simulink model "PV_system_modified"  (R2024a)
settings: Solver=VariableStepAuto  StartTime=0  StopTime=1.2  RelTol=1e-3
InitFcn:
  | PV_system_par;
undefined symbols (not defined in the file): Clink, D1, Delta, F_LL, F_LLG, F_LLLG, F_SLG, Fc, Fnom, I, Increment_MPPT, Ki_Ireg, Ki_VDCreg, Kp_Ireg, Kp_VDCreg, L1, L2, LimitL_Ireg, LimitL_VDCreg, Limits_MPPT, LimitU_Ireg, LimitU_VDCreg, P_load, Pnom, Pnom_xfo, Qc_load, Ql_load, RL, RLff, Ts_Control, Ts_Power, Vf, Vfd, Vnom_dc, Vnom_prim, Vnom_sec
libraries: spsThreePhaseParallelRLCLoadLib x5, spsThreePhaseFaultLib x4, spsSeriesRLCBranchLib x3, spsThreePhaseVIMeasurementLib x3, spsPMUPLLBasedPositiveSequenceLib x3, spsThreePhaseBreakerLib x3, spsThreePhaseTransformerTwoWindingsLib x2, slpidlib x2, spsabctodq0Lib x2, spsPowerPositiveSequenceLib x2, spsVoltageMeasurementLib x2, spsThreePhaseSourceLib x1
settings Model: Creator=MathWorks  LastModifiedBy=745
settings SolverCC: AlgebraicLoopSolver=TrustRegion
settings DataIOCC: FinalStateName=xFinal236  InitialState=xFinal236  LimitDataPoints=on  SaveFinalState=on  SaveFormat=Array  SignalLoggingSaveFormat=ModelDataLogs  SaveOutput=off  SignalLogging=off  DSMLogging=off  SaveTime=off  ReturnWorkspaceOutputs=off
settings OptimizationCC: ExpressionDepthLimit=2147483647  LifeSpan=inf
settings DebuggingCC: UnderspecifiedInitializationDetection=Classic  MergeDetectMultiDrivingBlocksExec=none  SolverPrmCheckMsg=warning  FcnCallInpInsideContextMsg=warning  UnconnectedInputMsg=warning  UnconnectedOutputMsg=warning  UnconnectedLineMsg=warning  StateNameClashWarn=warning  SFUnexpectedBacktrackingDiag=warning  SFNoUnconditionalDefaultTransitionDiag=warning  SFExecutionAtInitializationDiag=none  ArithmeticOperatorsInVariantConditions=warning
settings HardwareCC: ProdBitPerPointer=32  ProdBitPerSizeT=32  ProdBitPerPtrDiffT=32  ProdLargestAtomicFloat=None  ProdIntDivRoundTo=Undefined  ProdEndianess=Unspecified  ProdWordSize=32  ProdHWDeviceType=32-bit Generic
settings ModelReferenceCC: EnableRefExpFcnMdlSchedulingChecks=on  PropagateSignalLabelsOutOfModel=off
settings SFSimCC: SimUseLocalCustomCode=off  CustomCodeUndefinedFunction=UseInterfaceOnly
settings RTWCC: RTWUseLocalCustomCode=off  GPUComputeCapability=3.5
settings CodeAppCC: StateflowObjectComments=on
settings GRTTargetCC: TargetLangStandard=C89/C90 (ANSI)  CombineOutputUpdateFcns=off  GRTInterface=on
settings ConfigComp: CovMetricSettings=dw  CovSaveCumulativeToWorkspaceVar=on  CovSaveSingleToWorkspaceVar=on  CovExternalEMLEnable=off  CovSFcnEnable=off
settings SimscapeCC: SimscapeNormalizeSystem=off

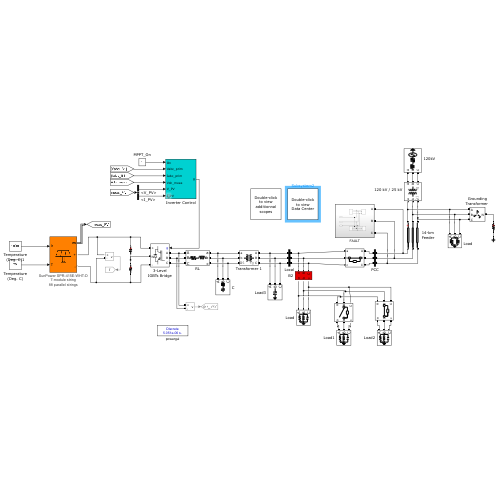
[thumbnail: Simulink's stored preview of the top-level diagram]
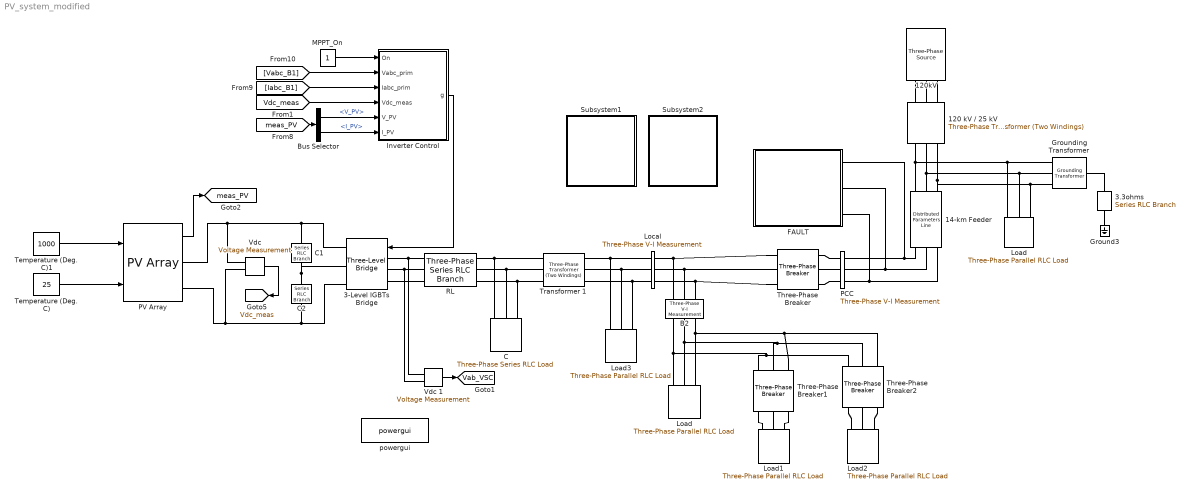
== system PV_system_modified ==
  " Load" : spsThreePhaseParallelRLCLoadLib/Three-Phase Parallel RLC Load  LConnTagsString=A|B|C  Configuration=Y (grounded)  NominalVoltage=Vnom_prim  Vabc=[1e3 1e3 1e3]  Vabcp=[1e3 1e3 1e3]  NominalFrequency=Fnom  UnbalancedPower=off  ActivePower=30e6  InductivePower=2e6  CapacitivePower=0  Pabc=[10e3 9e3 11e3]  QLabc=[100 90 110]  QCabc=[100 90 110]  Pabcp=[10e3 9e3 11e3]  QLabcp=[100 90 110]  QCabcp=[100 90 110]  Measurements=None  LoadType=constant Z
  "120 kV / 25 kV " : spsThreePhaseTransformerTwoWindingsLib/Three-Phase Transformer (Two Windings)  Winding1Connection=Yg  Winding2Connection=Delta (D1)  CoreType=Three single-phase transformers  SetSaturation=off  Hysteresis=off  DataFile='basic_model'  SetInitialFlux=off  Measurements=None  UNITS=pu  NominalPower=[47e6 Fnom ]  Winding1="[ 120e3  0.08/30   0.08 ]"  Winding2="[ Vnom_prim  0.08/30  0.08]"  Rm=500  Lm=500  L0=0.5  Saturation="[ 0,0  ;  0.005,1.2  ;  1.0,1.4 ]"  InitialFluxes=[ 0.8 , -0.8 , 0.7 ]  BreakLoop=off  DiscreteSolver=Trapezoidal iterative  DataType=off  TransfoNumber=0
  "120kV " : spsThreePhaseSourceLib/Three-Phase Source  InternalConnection=Yg  VoltagePhases=off  Voltage=(120000)*2.00543  PhaseAngle=-0.89585  Voltage_phases=[25e3 25e3 25e3]/sqrt(3)  PhaseAngles_phases=[0 -120 +120]  Frequency=Fnom  NonIdealSource=on  SpecifyImpedance=on  Resistance=0.8929  Inductance=16.58e-3  ShortCircuitLevel=2500e6  BaseVoltage=120e3  XRratio=7  BusType=swing  Pref=0  Qref=0  Prefabc=[10e3, 10e3, 10e3]  Qrefabc=[0, 0, 0]  Qmin=-inf  Qmax=inf
  14-km Feeder : spsDistributedParametersLineLib/Distributed Parameters Line  Phases=3  Length=14  Frequency=Fnom  Resistance=[0.1153 0.413]  Inductance=[1.05e-3 3.32e-3]  Capacitance=[11.33e-009 5.01e-009]  x1=[-6.06060606060606e-05 2.70356818258823e-09 -7448.2546576066 -48579.4518787537;-5.55555555555556e-05 2.70296987690159e-09 -7355.74615270988 -48593.5452588263;-5.05050505050505e-05 2.70236177241409e-09 -7263.21098177729 -48607.4624776782;-4.54545454545455e-05 2.70174387133024e-09 -7170.64948026713 -48621.2034848568;-4.04040404040404e-05 2.70111617589004e-09 -7078.06198373317 -48634.7682305481;-3.53535353535354e-05 2.70047868836901e-09 -6985.44882782342 -48648.1566655774;-3.03030303030303e-05 2.69983141107818e-09 -6892.81034827889 -48661.3687414089;-2.52525252525253e-05 2.69917434636406e-09 -6800.14688093242 -48674.4044101461;-2.02020202020202e-05 2.69850749660862e-09 -6707.45876170742 -48687.2636245322;-1.51515151515152e-05 2.69783086422934e-09 -6614.74632661666 -48699.94633795;-1.01010101010101e-05 2.69714445167914e-09 -6522.00991176108 -48712.4525044222;-5.05050505050505e-06 2.69644826144641e-09 -6429.24985332853 -48724.7820786115]  x2=[-6.06060606060606e-05 2.37344003803955e-09 -7561.18542903438 -48547.90625864;-5.55555555555556e-05 2.37275781583048e-09 -7468.73678212341 -48562.2147154482;-5.05050505050505e-05 2.37206699190463e-09 -7376.26105956317 -48576.3471246152;-4.54545454545455e-05 2.37136756876638e-09 -7283.75859659646 -48590.3034349081;-4.04040404040404e-05 2.37065954895129e-09 -7191.22972856301 -48604.0835957326;-3.53535353535354e-05 2.36994293502606e-09 -7098.67479089829 -48617.6875571329;-3.03030303030303e-05 2.36921772958855e-09 -7006.09411913227 -48631.115269792;-2.52525252525253e-05 2.36848393526779e-09 -6913.48804888821 -48644.3666850316;-2.02020202020202e-05 2.36774155472393e-09 -6820.85691588144 -48657.4417548129;-1.51515151515152e-05 2.36699059064823e-09 -6728.20105591817 -48670.340431736;-1.01010101010101e-05 2.3662310457631e-09 -6635.52080489422 -48683.0626690407;-5.05050505050505e-06 2.36546292282202e-09 -6542.81649879384 -48695.6084206065]  x3=[-6.06060606060606e-05 -1.40909290200934e-12 -26.0416127367686 -138.462500741439;-5.55555555555556e-05 -1.44156443022592e-12 -25.777933708129 -138.511832849198;-5.05050505050505e-05 -1.47403073248608e-12 -25.514161229377 -138.560662824145;-4.54545454545455e-05 -1.50649169109305e-12 -25.2502962567399 -138.60899048926;-4.04040404040404e-05 -1.53894718836944e-12 -24.9863397467807 -138.656815669347;-3.53535353535354e-05 -1.57139710665763e-12 -24.7222926563938 -138.704138191031;-3.03030303030303e-05 -1.60384132832025e-12 -24.4581559428022 -138.750957882757;-2.52525252525253e-05 -1.63627973574057e-12 -24.1939305635539 -138.797274574794;-2.02020202020202e-05 -1.66871221132296e-12 -23.929617476518 -138.843088099237;-1.51515151515152e-05 -1.70113863749325e-12 -23.6652176398819 -138.888398290001;-1.01010101010101e-05 -1.73355889669924e-12 -23.4007320121474 -138.933204982828;-5.05050505050505e-06 -1.76597287141107e-12 -23.1361615521271 -138.977508015286]  x4=[-6.06060606060606e-05 7.12180654461823e-12 -25.9634564564282 -178.876147541871;-5.55555555555556e-05 7.15742887638408e-12 -25.6228302123746 -178.925257586776;-5.05050505050505e-05 7.19302526105343e-12 -25.2821110804896 -178.973718992203;-4.54545454545455e-05 7.22859556958235e-12 -24.9413002959472 -179.021531582471;-4.04040404040404e-05 7.26413967302144e-12 -24.6003990942542 -179.068695184249;-3.53535353535354e-05 7.29965744251626e-12 -24.2594087112448 -179.115209626561;-3.03030303030303e-05 7.33514874930789e-12 -23.9183303830766 -179.161074740782;-2.52525252525253e-05 7.37061346473331e-12 -23.5771653462262 -179.206290360643;-2.02020202020202e-05 7.40605146022591e-12 -23.2359148374842 -179.250856322226;-1.51515151515152e-05 7.44146260731593e-12 -22.8945800939515 -179.294772463973;-1.01010101010101e-05 7.47684677763096e-12 -22.5531623530339 -179.338038626678;-5.05050505050505e-06 7.51220384289638e-12 -22.2116628524384 -179.380654653493]  x5=5.70973484498186e-05  V1=[0 0 0 2.512e-09 2.496e+04 2.496e+04;0 0 0 377 377 377;1.571 1.571 1.571 -1.525 -0.1391 -1.71]  V2=[0 0 0 2.184e-09 2.482e+04 2.482e+04;0 0 0 377 377 377;1.571 1.571 1.571 -1.563 -0.159 -1.73]  I1=[0 0 0 1.724e-11 7.342 7.342;0 0 0 377 377 377;1.571 1.571 1.571 0.451 3.099 1.528]  I2=[0 0 0 1.983e-11 170.2 170.2;0 0 0 377 377 377;1.571 1.571 1.571 -2.403 -0.1532 -1.724]  nHarmo=2  Measurements=None  Decoupling=off  VsMag0=0  VrMag0=0  VsAngle0=0  VrAngle0=0  IsMag0=0  IrMag0=0  IsAngle0=0  IrAngle0=0
      settings: LibrarySourceBlock=sps_lib/Power Grid Elements/Distributed Parameters Line
  3-Level IGBTs Bridge : spsThreeLevelBridgeLib/Three-Level Bridge  Arms=3  SnubberResistance=Rs  SbubberCapacitance=Cs  Device=IGBT / Diodes  Ron=Ron  ForwardVoltages="[  Vfd  Vf ]"  Measurements=None
      settings: AttributesFormatString=\n  LibrarySourceBlock=sps_lib/Power Electronics/Three-Level Bridge
  "3.3ohms " : spsSeriesRLCBranchLib/Series RLC Branch  LConnTagsString=__new0  RConnTagsString=__new0  BranchType=R  Resistance=3.3  Inductance=[]  SetiL0=off  InitialCurrent=0  Capacitance=[]  Setx0=off  InitialVoltage=0  Measurements=None
  B2 : spsThreePhaseVIMeasurementLib/Three-Phase V-I Measurement  VoltageMeasurement=phase-to-ground  SetLabelV=on  LabelV=Vabc_Load  Vpu=on  VpuLL=off  CurrentMeasurement=yes  SetLabelI=on  LabelI=Iabc_Load  Ipu=on  Pbase=250e3  Vbase=25e3  OutputType=Magnitude  PhasorSimulation=off  PSBequivalent=0
  Bus Selector : BusSelector  OutputSignals=V_PV,I_PV
  C : spsThreePhaseSeriesRLCLoadLib/Three-Phase Series RLC Load  LConnTagsString=A|B|C  Configuration=Delta  NominalVoltage=Vnom_sec  Vabc=[1e3 1e3 1e3]  Vabcp=[1e3 1e3 1e3]  NominalFrequency=Fnom  UnbalancedPower=off  ActivePower=Pc  InductivePower=0  CapacitivePower=Qc  Pabc=[10e3 9e3 11e3]  QLabc=[100 90 110]  QCabc=[100 90 110]  Pabcp=[10e3 9e3 11e3]  QLabcp=[100 90 110]  QCabcp=[100 90 110]  Measurements=None  LoadType=constant Z
  C1 : spsSeriesRLCBranchLib/Series RLC Branch  LConnTagsString=__new0  RConnTagsString=__new0  BranchType=C  Resistance=1.0  Inductance=1.0  SetiL0=off  InitialCurrent=0  Capacitance=Clink  Setx0=on  InitialVoltage=Vnom_dc/2  Measurements=None
  C2 : spsSeriesRLCBranchLib/Series RLC Branch  LConnTagsString=__new0  RConnTagsString=__new0  BranchType=C  Resistance=1.0  Inductance=1.0  SetiL0=off  InitialCurrent=0  Capacitance=Clink  Setx0=on  InitialVoltage=Vnom_dc/2  Measurements=None
  FAULT : Subsystem
  Ground3 : spsGroundLib/Ground  LConnTagsString=a
  "Grounding Transformer " : spsGroundingTransformerLib/Grounding Transformer   UNITS=pu  NominalPower="[100e6   Fnom]"  NominalVoltage=Vnom_prim  ZeroSequenceImpedance_pu=[0.025 0.75]  MagnetizationBranch_pu=[500 500]  ZeroSequenceImpedance_SI=[0.052083 589.05]  MagnetizationBranch_SI=[1041.7 3.927e+005]  Measurements=None
      settings: LibrarySourceBlock=|
      | sps_lib/Power Grid Elements/Grounding
      | Transformer
  Inverter Control : Subsystem  mask(Inverter Control){Pnom=Pnom, Fnom=Fnom, Vnom_prim=Vnom_prim, Vnom_sec=Vnom_sec, Vnom_dc=Vnom_dc, Increment_MPPT=Increment_MPPT, Limits_MPPT=Limits_MPPT, Vdc_ref_Init=Vnom_dc, Kp_VDCreg=Kp_VDCreg, Ki_VDCreg=Ki_VDCreg, Kp_Ireg=Kp_Ireg, Ki_Ireg=Ki_Ireg, RLff=RLff, Fc=Fc, Ts_Control=Ts_Control, Ts_PWMgenerator=Ts_Power}
      mask prompts: Pnom "Power (VA)"; Fnom "Frequency (Hz)"; Vnom_prim "Primary voltage (Vrms LL)"; Vnom_sec "Secondary voltage (Vrms LL)"; Vnom_dc "DC voltage (V)"; Increment_MPPT "Output increment (V)"; Limits_MPPT "Output limits [ Upper  Lower ]"; Vdc_ref_Init "Output initial value (V)"; Kp_VDCreg "Proportional gain"; Ki_VDCreg "Integral gain"; Kp_Ireg "Proportional gain"; Ki_Ireg "Integral gain"; RLff "Feedforward Values [Rff Lff]"; Fc "Carrier frequency (Hz)"; Ts_Control "Control systems"; Ts_PWMgenerator "PWM generator"
      mask help:
      | The main components of the Inverter Control are:
      | 1. PLL & Measurements
      | 2. Maximum Power Point Tracker System (MPPT) using a Perturb & Observe algorithm
      | 3. DC Voltage Regulator
      | 4. Current Regulator
      | 5. PWM Modulator
      mask DialogControl Container4 Prompt: Nominal Values:
      mask DialogControl Container3 Prompt: MPPT Controller:
      mask DialogControl Container8 Prompt: Dc Voltage Regulator:
      mask DialogControl Container6 Prompt: Current Regulator:
      mask DialogControl Container9 Prompt: PWM Modulator:
      mask DialogControl SampleTimes Prompt: Sample Times:
  Load : spsThreePhaseParallelRLCLoadLib/Three-Phase Parallel RLC Load  LConnTagsString=A|B|C  Configuration=Y (grounded)  NominalVoltage=Vnom_prim  Vabc=[1e3 1e3 1e3]  Vabcp=[1e3 1e3 1e3]  NominalFrequency=Fnom  UnbalancedPower=off  ActivePower=P_load*0.75  InductivePower=Ql_load*0.75  CapacitivePower=Qc_load*0.75  Pabc=[10e3 9e3 11e3]  QLabc=[100 90 110]  QCabc=[100 90 110]  Pabcp=[10e3 9e3 11e3]  QLabcp=[100 90 110]  QCabcp=[100 90 110]  Measurements=None  LoadType=constant Z
  Load1 : spsThreePhaseParallelRLCLoadLib/Three-Phase Parallel RLC Load  LConnTagsString=A|B|C  Configuration=Y (grounded)  NominalVoltage=Vnom_prim  Vabc=[1e3 1e3 1e3]  Vabcp=[1e3 1e3 1e3]  NominalFrequency=Fnom  UnbalancedPower=off  ActivePower=P_load*0.25  InductivePower=Ql_load*0.25  CapacitivePower=Qc_load*0.25  Pabc=[10e3 9e3 11e3]  QLabc=[100 90 110]  QCabc=[100 90 110]  Pabcp=[10e3 9e3 11e3]  QLabcp=[100 90 110]  QCabcp=[100 90 110]  Measurements=None  LoadType=constant Z
  Load2 : spsThreePhaseParallelRLCLoadLib/Three-Phase Parallel RLC Load  LConnTagsString=A|B|C  Configuration=Y (grounded)  NominalVoltage=Vnom_prim  Vabc=[1e3 1e3 1e3]  Vabcp=[1e3 1e3 1e3]  NominalFrequency=Fnom  UnbalancedPower=off  ActivePower=P_load*0.25  InductivePower=Ql_load*0.25  CapacitivePower=Qc_load*0.25  Pabc=[10e3 9e3 11e3]  QLabc=[100 90 110]  QCabc=[100 90 110]  Pabcp=[10e3 9e3 11e3]  QLabcp=[100 90 110]  QCabcp=[100 90 110]  Measurements=None  LoadType=constant Z
  Load3 : spsThreePhaseParallelRLCLoadLib/Three-Phase Parallel RLC Load  LConnTagsString=A|B|C  Configuration=Y (grounded)  NominalVoltage=Vnom_prim  Vabc=[1e3 1e3 1e3]  Vabcp=[1e3 1e3 1e3]  NominalFrequency=Fnom  UnbalancedPower=off  ActivePower=0  InductivePower=0  CapacitivePower=1  Pabc=[10e3 9e3 11e3]  QLabc=[100 90 110]  QCabc=[100 90 110]  Pabcp=[10e3 9e3 11e3]  QLabcp=[100 90 110]  QCabcp=[100 90 110]  Measurements=None  LoadType=constant Z
  Local : spsThreePhaseVIMeasurementLib/Three-Phase V-I Measurement  VoltageMeasurement=phase-to-ground  SetLabelV=on  LabelV=Vabc_Local  Vpu=on  VpuLL=off  CurrentMeasurement=yes  SetLabelI=on  LabelI=Iabc_Local  Ipu=on  Pbase=250e3  Vbase=25e3  OutputType=Magnitude  PhasorSimulation=off  PSBequivalent=0
  MPPT_On : Constant
  PCC : spsThreePhaseVIMeasurementLib/Three-Phase V-I Measurement  VoltageMeasurement=phase-to-ground  SetLabelV=on  LabelV=Vabc_PCC  Vpu=on  VpuLL=off  CurrentMeasurement=yes  SetLabelI=on  LabelI=Iabc_PCC  Ipu=on  Pbase=250e3  Vbase=25e3  OutputType=Magnitude  PhasorSimulation=off  PSBequivalent=0
  PV Array : spsPVArrayLib/PV Array  Npar=88  Nser=7  PlotType=array @ 1000 W/m2 & specified temperatures  S_vec="[ 1000  500  100 ]"  Temp_C_vec="[ 45 25  ]"  ModuleName=SunPower SPR-415E-WHT-D  PlotWhenSelected=off  Pm=414.801  Ncell=128  Voc=85.3  Isc=6.09  Vm=72.9  Im=5.69  beta_Voc_pc=-0.229  alpha_Isc_pc=0.030706  beta_Voc=-0.19534  alpha_Isc=0.00187  IL=6.0978  I0=7.1698e-13  nI=0.87223  Rsh=419.7781  Rs=0.53711  RobustModel=off  RobustCellTemperature=25  BAL=on  Tc=1e-6  Tfilter=5e-5
      settings: AttributesFormatString=|
      | %<ModuleName>
      | %<Nser>-module string
      | %<Npar> parallel strings
  RL : spsThreePhaseSeriesRLCBranchLib/Three-Phase Series RLC Branch  LConnTagsString=A|B|C  RConnTagsString=A|B|C  BranchType=RL  Resistance=RL(1)  Inductance=RL(2)  Capacitance=inf  Measurements=None
  Subsystem1 : Subsystem
      mask Display: disp('Double-click\nto view\nadditionnal\nscopes')
  Subsystem2 : Subsystem
      mask Display: disp('Double-click\nto view\nData Center')
  Temperature (Deg. C) : Constant  Value=25
  Temperature (Deg. C)1 : Constant  Value=1000
  Three-Phase Breaker : spsThreePhaseBreakerLib/Three-Phase Breaker  InitialState=closed  SwitchA=on  SwitchB=on  SwitchC=on  SwitchTimes=[0.5+I 1.5+I]  External=off  BreakerResistance=0.01  SnubberResistance=1e6  SnubberCapacitance=inf  Measurements=None
  Three-Phase Breaker1 : spsThreePhaseBreakerLib/Three-Phase Breaker  InitialState=open  SwitchA=on  SwitchB=on  SwitchC=on  SwitchTimes=[0.5+L1 1.5+L1]  External=off  BreakerResistance=0.01  SnubberResistance=1e6  SnubberCapacitance=inf  Measurements=None
  Three-Phase Breaker2 : spsThreePhaseBreakerLib/Three-Phase Breaker  InitialState=closed  SwitchA=on  SwitchB=on  SwitchC=on  SwitchTimes=[0.5+L2 1.5+L2]  External=off  BreakerResistance=0.01  SnubberResistance=1e6  SnubberCapacitance=inf  Measurements=None
  Transformer 1 : spsThreePhaseTransformerTwoWindingsLib/Three-Phase Transformer (Two Windings)  Winding1Connection=Yg  Winding2Connection=Delta (D1)  CoreType=Three single-phase transformers  SetSaturation=off  Hysteresis=off  DataFile='hysteresis'  SetInitialFlux=off  Measurements=None  UNITS=pu  NominalPower=[Pnom_xfo, Fnom ]  Winding1=W1_xfo  Winding2=W2_xfo  Rm=Rm_xfo  Lm=Lm_xfo  L0=0.5  Saturation=[ 0,0 ; 0.0024,1.2 ; 1.0,1.52 ]  InitialFluxes=[ 0.8 , -0.8 , 0.7 ]  BreakLoop=off  DiscreteSolver=Trapezoidal iterative  DataType=off  TransfoNumber=0
  "Vdc " : spsVoltageMeasurementLib/Voltage Measurement  Tag=PoWeRsYsTeMmEaSuReMeNt  PhasorSimulation=off  OutputType=Magnitude  PSBequivalent=0
  Vdc 1 : spsVoltageMeasurementLib/Voltage Measurement  Tag=PoWeRsYsTeMmEaSuReMeNt  PhasorSimulation=off  OutputType=Magnitude  PSBequivalent=0
  powergui : sps_lib/powergui  Priority=1  SimulationMode=Discrete  SampleTime=Ts_Power  frequency=60  Iterations=50  frequencyindice=0  Pbase=100e6  ErrMax=0.0001  UnitsV=kV  UnitsW=MW  buscounter=0  FunctionMessages=off  echomessages=off  EnableUseOfTLC=off  CurrentSourceSwitches=off  DisableSnubberDevices=off  DisableRonSwitches=off  DisableVfSwitches=off  DisplayEquations=off  AutomaticDiscreteSolvers=off  SolverType=Tustin  Interpol=off  ExternalGateDelay=off  methode=off  Ts=0  x0status=blocks  SPID=off  SwTol=0  HookPort=off  NonlinearTolerance=1e-4  nMaxIteration=15  ContinueOnMaxIteration=off  RestoreLinks=warning  ResistiveCurrentMeasurement=off  Frange=[0:2:500]  Ylog=off  Xlog=on  ShowGrid=off  save=off  variable=ZData  structure=VaIa_Grid  ZoomFFT=off  StartTime=1.4  cycles=3  DisplayStyle=1  fundamental=60  FreqAxis=on  MaxFrequency=5000  frequencyindicesteady=1  RmsSteady=1  display=off
  tag scope: Vab_VSC=global, Vdc_meas=global, meas_PV=global
  wires:
  Vdc 1/1 -> [Vab_VSC]
  PV Array/1 -> [meas_PV]
  Inverter Control/1(g) -> 3-Level IGBTs Bridge/1
  [Vabc_B1] -> Inverter Control/2(Vabc_prim)
  [Iabc_B1] -> Inverter Control/3(Iabc_prim)
  [Vdc_meas] -> Inverter Control/4(Vdc_meas)
  [meas_PV] -> Bus Selector/1
  "Vdc "/1 -> [Vdc_meas]
  Bus Selector/1 -> Inverter Control/5(V_PV)  "<V_PV>"
  Bus Selector/2 -> Inverter Control/6(I_PV)  "<I_PV>"
  MPPT_On/1 -> Inverter Control/1(On)
  Temperature (Deg. C)/1 -> PV Array/2
  Temperature (Deg. C)1/1 -> PV Array/1
  connections:
  Local/LConn1 -- Load3/LConn1 -- Transformer 1/LConn1
  Local/LConn2 -- Load3/LConn2 -- Transformer 1/LConn2
  Local/LConn3 -- Transformer 1/LConn3 -- Load3/LConn3
  C2/LConn1 -- 3-Level IGBTs Bridge/RConn2 -- C1/RConn1
  C1/LConn1 -- PV Array/RConn1 -- "Vdc "/LConn1 -- 3-Level IGBTs Bridge/RConn1
  C2/RConn1 -- PV Array/RConn2 -- "Vdc "/LConn2 -- 3-Level IGBTs Bridge/RConn3
  RL/LConn1 -- Vdc 1/LConn1 -- 3-Level IGBTs Bridge/LConn1
  RL/LConn2 -- Vdc 1/LConn2 -- 3-Level IGBTs Bridge/LConn2
  RL/LConn3 -- 3-Level IGBTs Bridge/LConn3
  C/LConn1 -- Transformer 1/RConn1 -- RL/RConn1
  C/LConn2 -- Transformer 1/RConn2 -- RL/RConn2
  C/LConn3 -- Transformer 1/RConn3 -- RL/RConn3
  "Grounding Transformer "/RConn1 -- "3.3ohms "/LConn1
  "3.3ohms "/RConn1 -- Ground3/LConn1
  "120 kV / 25 kV "/RConn1 -- 14-km Feeder/LConn1 -- " Load"/LConn1 -- "Grounding Transformer "/LConn1
  "120 kV / 25 kV "/RConn2 -- " Load"/LConn2 -- "Grounding Transformer "/LConn2 -- 14-km Feeder/LConn2
  "120 kV / 25 kV "/RConn3 -- " Load"/LConn3 -- "Grounding Transformer "/LConn3 -- 14-km Feeder/LConn3
  "120kV "/RConn1 -- "120 kV / 25 kV "/LConn1
  "120kV "/RConn2 -- "120 kV / 25 kV "/LConn2
  "120kV "/RConn3 -- "120 kV / 25 kV "/LConn3
  B2/LConn1 -- Local/RConn1 -- Three-Phase Breaker/RConn1
  Load/LConn2 -- Three-Phase Breaker2/LConn2 -- Three-Phase Breaker1/LConn2 -- B2/RConn2
  B2/RConn1 -- Three-Phase Breaker2/LConn1 -- Three-Phase Breaker1/LConn1 -- Load/LConn1
  Load/LConn3 -- Three-Phase Breaker2/LConn3 -- Three-Phase Breaker1/LConn3 -- B2/RConn3
  Local/RConn2 -- Three-Phase Breaker/RConn2 -- B2/LConn2
  Local/RConn3 -- Three-Phase Breaker/RConn3 -- B2/LConn3
  Three-Phase Breaker1/RConn3 -- Load1/LConn3
  Three-Phase Breaker1/RConn2 -- Load1/LConn2
  Three-Phase Breaker1/RConn1 -- Load1/LConn1
  Load2/LConn1 -- Three-Phase Breaker2/RConn1
  Load2/LConn2 -- Three-Phase Breaker2/RConn2
  Load2/LConn3 -- Three-Phase Breaker2/RConn3
  PCC/LConn2 -- Three-Phase Breaker/LConn2
  PCC/LConn1 -- Three-Phase Breaker/LConn1
  PCC/LConn3 -- Three-Phase Breaker/LConn3
  14-km Feeder/RConn1 -- PCC/RConn1 -- FAULT/LConn1
  14-km Feeder/RConn2 -- PCC/RConn2 -- FAULT/LConn2
  14-km Feeder/RConn3 -- FAULT/LConn3 -- PCC/RConn3

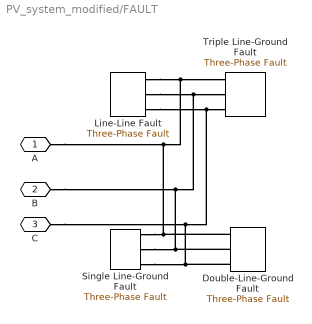
== system PV_system_modified/FAULT ==
  Double-Line-Ground Fault : spsThreePhaseFaultLib/Three-Phase Fault  InitialStates=0  FaultA=on  FaultB=on  FaultC=off  GroundFault=on  SwitchTimes=[0.5+F_LLG 0.6+F_LLG]  External=off  SwitchStatus=NaN  FaultResistance=Rf  GroundResistance=Rg  SnubberResistance=1e6  SnubberCapacitance=inf  Measurements=None
  Line-Line Fault : spsThreePhaseFaultLib/Three-Phase Fault  InitialStates=0  FaultA=on  FaultB=on  FaultC=off  GroundFault=off  SwitchTimes=[0.5+F_LL 0.6+F_LL]  External=off  SwitchStatus=NaN  FaultResistance=Rf  GroundResistance=0.01  SnubberResistance=1e6  SnubberCapacitance=inf  Measurements=None
  Single Line-Ground Fault : spsThreePhaseFaultLib/Three-Phase Fault  InitialStates=0  FaultA=on  FaultB=off  FaultC=off  GroundFault=on  SwitchTimes=[0.5+F_SLG 0.6+F_SLG]  External=off  SwitchStatus=NaN  FaultResistance=Rf  GroundResistance=Rg  SnubberResistance=1e6  SnubberCapacitance=inf  Measurements=None
  Triple Line-Ground Fault : spsThreePhaseFaultLib/Three-Phase Fault  InitialStates=0  FaultA=on  FaultB=on  FaultC=on  GroundFault=on  SwitchTimes=[0.5+F_LLLG 0.6+F_LLLG]  External=off  SwitchStatus=NaN  FaultResistance=Rf  GroundResistance=Rg  SnubberResistance=1e6  SnubberCapacitance=inf  Measurements=None
  A : PMIOPort  Side=Left
  B : PMIOPort  Port=2  Side=Left
  C : PMIOPort  Port=3  Side=Left
  connections:
  Line-Line Fault/LConn1 -- Double-Line-Ground Fault/LConn1 -- Single Line-Ground Fault/LConn1 -- A/RConn1 -- Triple Line-Ground Fault/LConn1
  Line-Line Fault/LConn2 -- Double-Line-Ground Fault/LConn2 -- Single Line-Ground Fault/LConn2 -- B/RConn1 -- Triple Line-Ground Fault/LConn2
  Line-Line Fault/LConn3 -- Double-Line-Ground Fault/LConn3 -- Single Line-Ground Fault/LConn3 -- C/RConn1 -- Triple Line-Ground Fault/LConn3

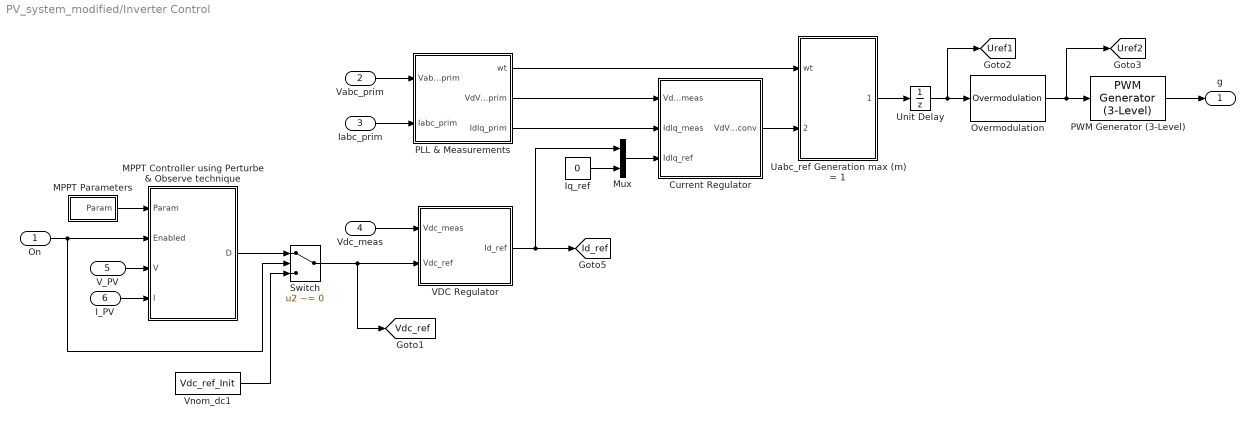
== system PV_system_modified/Inverter Control ==
  On : Inport  PortDimensions=1
  Vabc_prim : Inport  Port=2  PortDimensions=3
  Iabc_prim : Inport  Port=3  PortDimensions=3
  Vdc_meas : Inport  Port=4  PortDimensions=1
  V_PV : Inport  Port=5  PortDimensions=1
  I_PV : Inport  Port=6  PortDimensions=1
  Current Regulator : Subsystem
  Iq_ref : Constant  Value=0
  MPPT Parameters : Subsystem
  "MPPT Controller using Perturbe & Observe technique " : MATLAB Function  TreatAsAtomicUnit=on
  Mux : Mux  Inputs=2
  Overmodulation : spsOvermodulationLib/Overmodulation  OverModType=Flat top
      settings: LibrarySourceBlock=sps_lib/Power Electronics/Power Electronics Control/Overmodulation
  PLL & Measurements : Subsystem
  PWM Generator (3-Level) : spsPWMGenerator3LevelLib/PWM Generator (3-Level)  ModulatorType=Three-phase bridge (12 pulses)  ModulatorMode=Unsynchronized  nF=27  Fc=Fc  ModulatingSignals=off  m=0.8  Freq=60  Phase=0  Ts=Ts_PWMgenerator
      settings: LibrarySourceBlock=|
      | sps_lib/Power Electronics/Power Electronics Control/PWM Generator
      | (3-Level)
  Switch : Switch  Criteria=u2 ~= 0  SaturateOnIntegerOverflow=off  InputSameDT=off
  Uabc_ref Generation max (m) = 1 : Subsystem
  Unit Delay : UnitDelay  SampleTime=Ts_Control  HasFrameUpgradeWarning=on
  VDC Regulator : Subsystem
  Vnom_dc1 : Constant  Value=Vdc_ref_Init
  g : Outport  VectorParamsAs1DForOutWhenUnconnected=off
  tag scope: Id_ref=global, Uref1=global, Uref2=global, Vdc_ref=global
  wires:
  PLL & Measurements/1(wt) -> Uabc_ref Generation max (m) = 1/1(wt)
  Current Regulator/1(VdVq_conv) -> Uabc_ref Generation max (m) = 1/2(VdVq_conv)
  Iq_ref/1 -> Mux/2
  Mux/1 -> Current Regulator/3(IdIq_ref)
  PLL & Measurements/3(IdIq_prim) -> Current Regulator/2(IdIq_meas)
  PLL & Measurements/2(VdVq_prim) -> Current Regulator/1(VdVq_meas)
  Vabc_prim/1 -> PLL & Measurements/1(Vabc_prim)
  Iabc_prim/1 -> PLL & Measurements/2(Iabc_prim)
  PWM Generator (3-Level)/1 -> g/1
  Vdc_meas/1 -> VDC Regulator/1(Vdc_meas)
  VDC Regulator/1(Id_ref) -> [Id_ref], Mux/1
  V_PV/1 -> "MPPT Controller using Perturbe & Observe technique "/3(V)
  I_PV/1 -> "MPPT Controller using Perturbe & Observe technique "/4(I)
  MPPT Parameters/1(Param) -> "MPPT Controller using Perturbe & Observe technique "/1(Param)
  On/1 -> "MPPT Controller using Perturbe & Observe technique "/2(Enabled), Switch/2
  Overmodulation/1 -> [Uref2], PWM Generator (3-Level)/1
  Unit Delay/1 -> [Uref1], Overmodulation/1
  "MPPT Controller using Perturbe & Observe technique "/1(D) -> Switch/1
  Switch/1 -> [Vdc_ref], VDC Regulator/2(Vdc_ref)
  Vnom_dc1/1 -> Switch/3
  Uabc_ref Generation max (m) = 1/1(Uabc_ref) -> Unit Delay/1

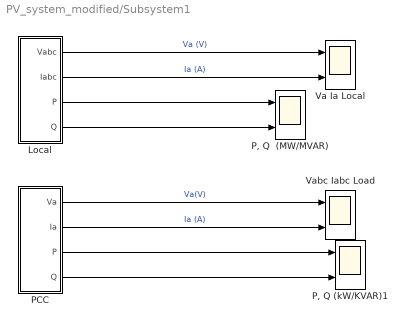
== system PV_system_modified/Subsystem1 ==
  Local : Subsystem
  "P, Q  (MW/MVAR)" : Scope  NumInputPorts=2
  "P, Q (kW/KVAR)1" : Scope  NumInputPorts=2
  PCC : Subsystem
  Va Ia Local : Scope  NumInputPorts=2
  Vabc Iabc Load : Scope  NumInputPorts=2
  wires:
  Local/3(P) -> "P, Q  (MW/MVAR)"/1
  Local/1(Vabc) -> Va Ia Local/1  "Va (V)"
  PCC/2(Ia) -> Vabc Iabc Load/2  "Ia (A)"
  PCC/4(Q) -> "P, Q (kW/KVAR)1"/2
  PCC/3(P) -> "P, Q (kW/KVAR)1"/1
  PCC/1(Va) -> Vabc Iabc Load/1  "Va(V)"
  Local/2(Iabc) -> Va Ia Local/2  "Ia (A)"
  Local/4(Q) -> "P, Q  (MW/MVAR)"/2

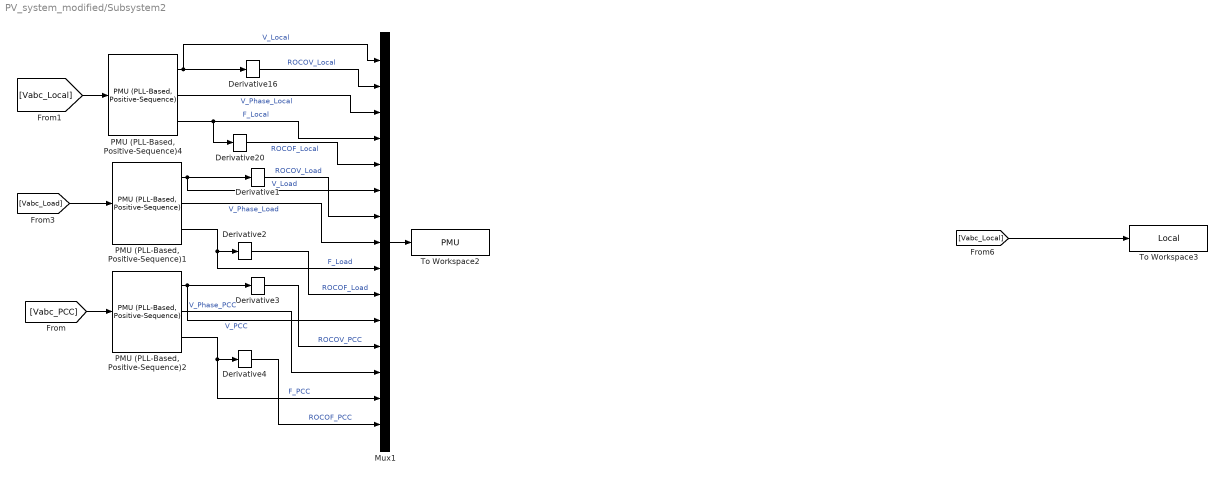
== system PV_system_modified/Subsystem2 ==
  Derivative{1..4,16,20} (6 alike) : Derivative
  Mux1 : Mux  Inputs=15
  "PMU (PLL-Based, Positive-Sequence)1" : spsPMUPLLBasedPositiveSequenceLib/PMU (PLL-Based, Positive-Sequence)  nominalFrequency=60  samplingRate=64  reportingFactor=1
      settings: LibrarySourceBlock=|
      | sps_lib/Sensors and Measurements/PMU
      | (PLL-Based,
      | Positive-Sequence)
  "PMU (PLL-Based, Positive-Sequence)2" : spsPMUPLLBasedPositiveSequenceLib/PMU (PLL-Based, Positive-Sequence)  nominalFrequency=60  samplingRate=64  reportingFactor=1
      settings: LibrarySourceBlock=|
      | sps_lib/Sensors and Measurements/PMU
      | (PLL-Based,
      | Positive-Sequence)
  "PMU (PLL-Based, Positive-Sequence)4" : spsPMUPLLBasedPositiveSequenceLib/PMU (PLL-Based, Positive-Sequence)  nominalFrequency=60  samplingRate=64  reportingFactor=1
      settings: LibrarySourceBlock=|
      | sps_lib/Sensors and Measurements/PMU
      | (PLL-Based,
      | Positive-Sequence)
  To Workspace2 : ToWorkspace  VariableName=PMU  SampleTime=1/60
      settings: Save2DSignal=2-D array (concatenate along first dimension)
  To Workspace3 : ToWorkspace  VariableName=Local  SampleTime=1/60/64
      settings: Save2DSignal=2-D array (concatenate along first dimension)
  wires:
  Derivative16/1 -> Mux1/2  "ROCOV_Local"
  "PMU (PLL-Based, Positive-Sequence)4"/1 -> Mux1/1, Derivative16/1  "V_Local"
  Mux1/1 -> To Workspace2/1
  "PMU (PLL-Based, Positive-Sequence)4"/2 -> Mux1/3  "V_Phase_Local"
  "PMU (PLL-Based, Positive-Sequence)4"/3 -> Mux1/4, Derivative20/1  "F_Local"
  Derivative20/1 -> Mux1/5  "ROCOF_Local"
  [Vabc_Local] -> "PMU (PLL-Based, Positive-Sequence)4"/1
  [Vabc_Local] -> To Workspace3/1
  [Vabc_Load] -> "PMU (PLL-Based, Positive-Sequence)1"/1
  Derivative2/1 -> Mux1/10  "ROCOF_Load"
  "PMU (PLL-Based, Positive-Sequence)1"/3 -> Mux1/9, Derivative2/1  "F_Load"
  "PMU (PLL-Based, Positive-Sequence)1"/2 -> Mux1/8  "V_Phase_Load"
  "PMU (PLL-Based, Positive-Sequence)1"/1 -> Mux1/6, Derivative1/1  "V_Load"
  Derivative1/1 -> Mux1/7  "ROCOV_Load"
  Derivative3/1 -> Mux1/12  "ROCOV_PCC"
  "PMU (PLL-Based, Positive-Sequence)2"/1 -> Mux1/11, Derivative3/1  "V_PCC"
  "PMU (PLL-Based, Positive-Sequence)2"/2 -> Mux1/13  "V_Phase_PCC"
  "PMU (PLL-Based, Positive-Sequence)2"/3 -> Mux1/14, Derivative4/1  "F_PCC"
  Derivative4/1 -> Mux1/15  "ROCOF_PCC"
  [Vabc_PCC] -> "PMU (PLL-Based, Positive-Sequence)2"/1

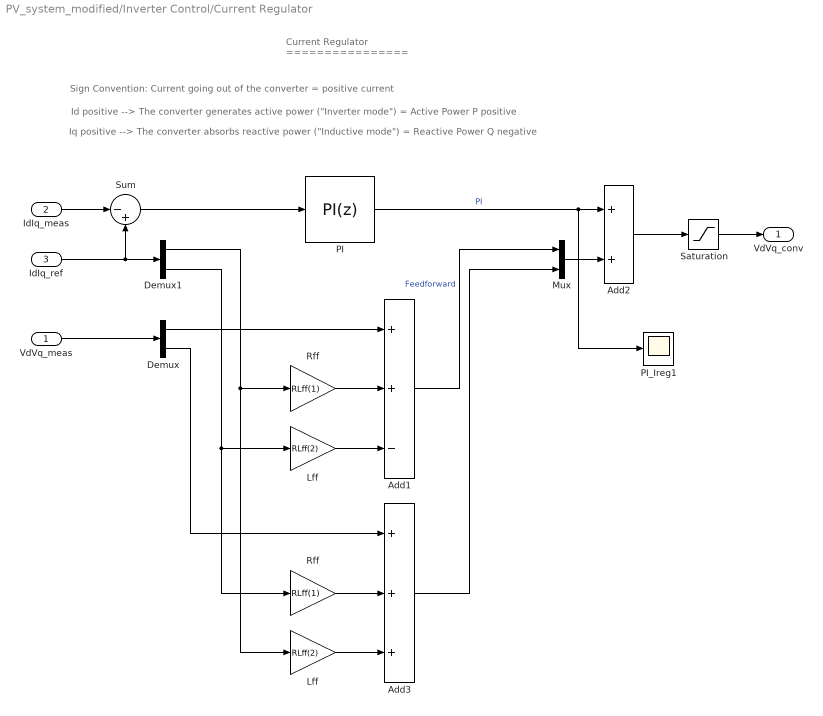
== system PV_system_modified/Inverter Control/Current Regulator ==
  note: Current Regulator
      | ================
  note: Sign Convention: Current going out of the converter = positive current
  note: Iq positive --> The converter absorbs reactive power ("Inductive mode") = Reactive Power Q negative
  note: Id positive --> The converter generates active power ("Inverter mode") = Active Power P positive
  VdVq_meas : Inport  PortDimensions=2
  IdIq_meas : Inport  Port=2  PortDimensions=2
  IdIq_ref : Inport  Port=3  PortDimensions=2
  Add1 : Sum  Inputs=++-
  Add2 : Sum
  Add3 : Sum  Inputs=+++
  Demux : Demux  Outputs=2
  Demux1 : Demux  Outputs=2
  Lff : Gain  Gain=RLff(2)  SaturateOnIntegerOverflow=on  OutDataTypeStr=Inherit: Same as input  ParamDataTypeStr=Inherit: Same as input
  "Lff  " : Gain  Gain=RLff(2)  SaturateOnIntegerOverflow=on  OutDataTypeStr=Inherit: Same as input  ParamDataTypeStr=Inherit: Same as input
  Mux : Mux  Inputs=2
  PI : slpidlib/PID Controller  Controller=PI  Form=Parallel  TimeDomain=Discrete-time  UseExternalTs=off  SampleTime=Ts_Control  IntegratorMethod=Forward Euler  FilterMethod=Forward Euler  ControllerParametersSource=internal  P=Kp_Ireg  I=Ki_Ireg  UseKiTs=off  D=0  UseExternalDerivativeSource=off  N=100  UseFilter=on  TunerSelectOption=Transfer Function Based (PID Tuner App)  InitialConditionSource=internal  InitialConditionForIntegrator=0  InitialConditionForFilter=0  DifferentiatorICPrevScaledInput=0  ExternalReset=none  TrackingMode=off  Kt=1  LimitOutput=on  SatLimitsSource=internal  UpperSaturationLimit=LimitU_Ireg  LowerSaturationLimit=LimitL_Ireg  LinearizeAsGain=off  AntiWindupMode=none  Kb=1  LimitIntegrator=off  UpperIntegratorSaturationLimit=inf  LowerIntegratorSaturationLimit=-inf  POutMin=[]  POutMax=[]  IOutMin=[]  IOutMax=[]  DOutMin=[]  DOutMax=[]  NOutMin=[]  NOutMax=[]  SumOutMin=[]  SumOutMax=[]  SaturationOutMin=[]  SaturationOutMax=[]  PParamMin=[]  PParamMax=[]  IParamMin=[]  IParamMax=[]  DParamMin=[]  DParamMax=[]  NParamMin=[]  NParamMax=[]  KbParamMin=[]  KbParamMax=[]  KtParamMin=[]  KtParamMax=[]  KbOutMin=[]  KbOutMax=[]  KtOutMin=[]  KtOutMax=[]  IntegratorOutMin=[]  IntegratorOutMax=[]  FilterOutMin=[]  FilterOutMax=[]  SumI1OutMin=[]  SumI1OutMax=[]  SumI2OutMin=[]  SumI2OutMax=[]  SumI3OutMin=[]  SumI3OutMax=[]  SumI4OutMin=[]  SumI4OutMax=[]  SumDOutMin=[]  SumDOutMax=[]  DifferentiatorOutMin=[]  DifferentiatorOutMax=[]  FilterDiffOutCoefMin=[]  FilterDiffOutCoefMax=[]  ReciprocalOutMin=[]  ReciprocalOutMax=[]  SumDenOutMin=[]  SumDenOutMax=[]  SumNumOutMin=[]  SumNumOutMax=[]  DivideOutMin=[]  DivideOutMax=[]  UdiffTsProdOutMin=[]  UdiffTsProdOutMax=[]  NTsProdOutMin=[]  NTsProdOutMax=[]  UintegralTsProdOutMin=[]  UintegralTsProdOutMax=[]  UngainTsProdOutMin=[]  UngainTsProdOutMax=[]  ClampingZeroOutDataTypeStr=Inherit: Inherit via back propagation  ClampingZeroOutMin=[]  ClampingZeroOutMax=[]  FilterDenConstantOutDataTypeStr=Inherit: Inherit via back propagation  FilterDenConstantOutMin=[]  FilterDenConstantOutMax=[]  PCopyOutDataTypeStr=Inherit: Inherit via back propagation  PCopyOutMin=[]  PCopyOutMax=[]  NCopyOutDataTypeStr=Inherit: Inherit via back propagation  NCopyOutMin=[]  NCopyOutMax=[]  IntegratorContinuousStateAttributes=''  IntegratorStateMustResolveToSignalObject=off  IntegratorRTWStateStorageClass=Auto  FilterContinuousStateAttributes=''  FilterStateMustResolveToSignalObject=off  FilterRTWStateStorageClass=Auto  ParallelPVariant=InternalParameters  IdealPVariant=Disabled  IVariant=InternalParameters  DVariant=Disabled  IntegratorVariant=Discrete  SatVariant=Enabled  AWVariant=Passthrough  PCopyVariant=Disabled  TRVariant=Disabled  FdbkBlocksVariant=Forward  IdealPFdbkVariant=Disabled  SatFdbkVariant=Disabled  DerivativeFilterVariant=Disabled  NVariant=Disabled  NCopyVariant=Disabled_SignalSpec  FilterICVariant=Disabled  IntegratorICVariant=InternalICs  ExternalResetVariant=Disabled  TRSumVariant=Passthrough  SumFdbkVariant=Disabled  SumVariant=Sum_PI  TsampFilterVariant=InternalTs  TsampNgainVariant=Passthrough  TsampIntegralVariant=Disabled_SignalSpec  ExternalSaturationOutDataTypeStr=Inherit: Same as second input  DerivativeSourceVariant=Disabled
  PI_Ireg1 : Scope
  Rff : Gain  Gain=RLff(1)  SaturateOnIntegerOverflow=on  OutDataTypeStr=Inherit: Same as input  ParamDataTypeStr=Inherit: Same as input
  "Rff " : Gain  Gain=RLff(1)  SaturateOnIntegerOverflow=on  OutDataTypeStr=Inherit: Same as input  ParamDataTypeStr=Inherit: Same as input
  Saturation : Saturate  UpperLimit=LimitU_Ireg  LowerLimit=LimitL_Ireg
  Sum : Sum  Inputs=|-+
  VdVq_conv : Outport  VectorParamsAs1DForOutWhenUnconnected=off
  wires:
  Mux/1 -> Add2/2
  PI/1 -> PI_Ireg1/1, Add2/1  "PI"
  Sum/1 -> PI/1
  IdIq_ref/1 -> Sum/2, Demux1/1
  IdIq_meas/1 -> Sum/1
  Add2/1 -> Saturation/1
  Saturation/1 -> VdVq_conv/1
  VdVq_meas/1 -> Demux/1
  Demux/1 -> Add1/1
  "Rff "/1 -> Add1/2
  Demux1/1 -> "Rff "/1, Lff/1
  "Lff  "/1 -> Add1/3
  Demux1/2 -> "Lff  "/1, Rff/1
  Rff/1 -> Add3/2
  Lff/1 -> Add3/3
  Add1/1 -> Mux/1  "Feedforward"
  Demux/2 -> Add3/1
  Add3/1 -> Mux/2

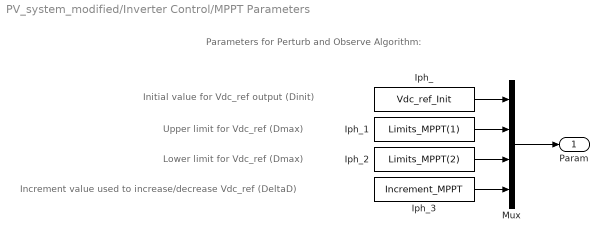
== system PV_system_modified/Inverter Control/MPPT Parameters ==
  note: Parameters for Perturb and Observe Algorithm:
  note: Lower limit for Vdc_ref (Dmax)
  note: Initial value for Vdc_ref output (Dinit)
  note: Increment value used to increase/decrease Vdc_ref (DeltaD)
  note: Upper limit for Vdc_ref (Dmax)
  Iph_ : Constant  Value=Vdc_ref_Init
  Iph_1 : Constant  Value=Limits_MPPT(1)
  Iph_2 : Constant  Value=Limits_MPPT(2)
  Iph_3 : Constant  Value=Increment_MPPT
  Mux : Mux
  Param : Outport  VectorParamsAs1DForOutWhenUnconnected=off
  wires:
  Mux/1 -> Param/1
  Iph_3/1 -> Mux/4
  Iph_2/1 -> Mux/3
  Iph_1/1 -> Mux/2
  Iph_/1 -> Mux/1

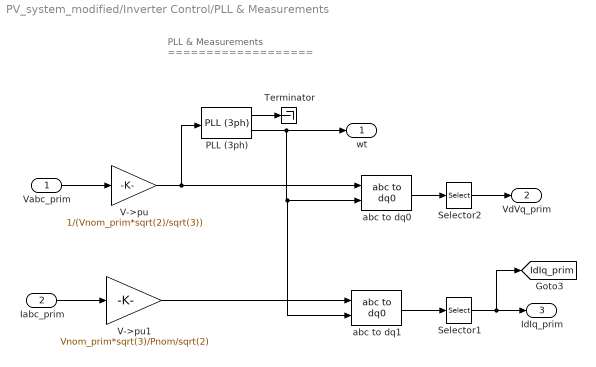
== system PV_system_modified/Inverter Control/PLL & Measurements ==
  note: PLL & Measurements
      | ===================
  Vabc_prim : Inport
  Iabc_prim : Inport  Port=2
  PLL (3ph) : spsPLL3phLib/PLL (3ph)  Fmin=45  Par_Init="[-0.57  Fnom]"  ParK=[180, 3200, 1]  TcD=1e-4  MaxRateChangeFreq=12  FilterCutOffFreq=25  Ts=Ts_Control  AGC=on
  Selector1 : Selector  InputPortWidth=3  IndexOptions=Index vector (dialog)  Indices=[1 2]  OutputSizes=1
  Selector2 : Selector  InputPortWidth=3  IndexOptions=Index vector (dialog)  Indices=[1 2]  OutputSizes=1
  Terminator : Terminator
  V->pu : Gain  Gain=1/(Vnom_prim*sqrt(2)/sqrt(3))  SaturateOnIntegerOverflow=on  OutDataTypeStr=Inherit: Same as input  ParamDataTypeStr=Inherit: Same as input
  V->pu1 : Gain  Gain=Vnom_prim*sqrt(3)/Pnom/sqrt(2)  SaturateOnIntegerOverflow=on  OutDataTypeStr=Inherit: Same as input  ParamDataTypeStr=Inherit: Same as input
  abc to dq0 : spsabctodq0Lib/abc to dq0  Alignment=90 degrees behind phase A axis
  abc to dq1 : spsabctodq0Lib/abc to dq0  Alignment=90 degrees behind phase A axis
  wt : Outport  VectorParamsAs1DForOutWhenUnconnected=off
  VdVq_prim : Outport  Port=2  VectorParamsAs1DForOutWhenUnconnected=off
  IdIq_prim : Outport  Port=3  VectorParamsAs1DForOutWhenUnconnected=off
  tag scope: IdIq_prim=global
  wires:
  V->pu1/1 -> abc to dq1/1
  V->pu/1 -> PLL (3ph)/1, abc to dq0/1
  abc to dq1/1 -> Selector1/1
  Vabc_prim/1 -> V->pu/1
  Iabc_prim/1 -> V->pu1/1
  abc to dq0/1 -> Selector2/1
  Selector2/1 -> VdVq_prim/1
  Selector1/1 -> [IdIq_prim], IdIq_prim/1
  PLL (3ph)/2 -> wt/1, abc to dq1/2, abc to dq0/2
  PLL (3ph)/1 -> Terminator/1

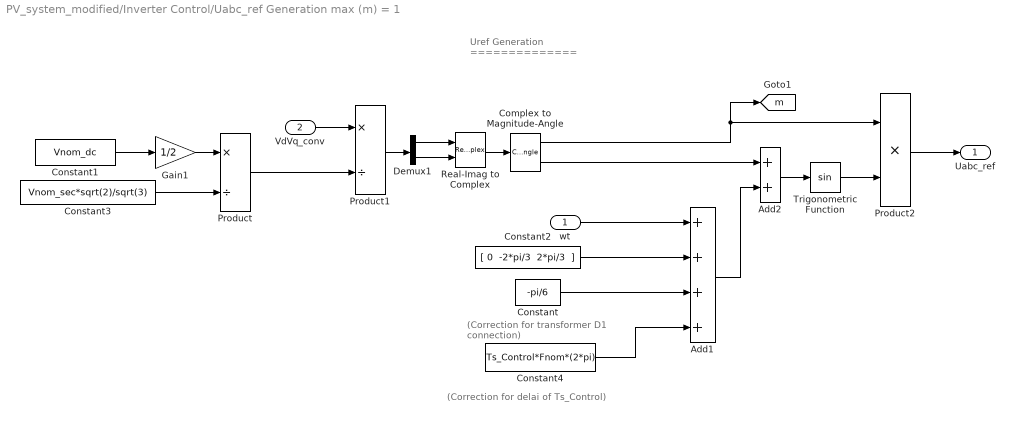
== system PV_system_modified/Inverter Control/Uabc_ref Generation max (m) = 1 ==
  note: (Correction for transformer
      |  D1 connection)
  note: (Correction for delai of Ts_Control)
  note: Uref Generation
      | ==============
  wt : Inport
  VdVq_conv : Inport  Port=2
  Add1 : Sum  Inputs=++++
  Add2 : Sum
  Complex to Magnitude-Angle : ComplexToMagnitudeAngle
  Constant : Constant  Value=-pi/6
  Constant1 : Constant  Value=Vnom_dc
  Constant2 : Constant  Value="[ 0  -2*pi/3  2*pi/3  ]"
  Constant3 : Constant  Value=Vnom_sec*sqrt(2)/sqrt(3)
  Constant4 : Constant  Value=Ts_Control*Fnom*(2*pi)
  Demux1 : Demux  Outputs=2
  Gain1 : Gain  Gain=1/2
  Product : Product  Inputs=*/  RndMeth=Zero
  Product1 : Product  Inputs=*/  RndMeth=Zero
  Product2 : Product  Inputs=**  RndMeth=Zero
  Real-Imag to Complex : RealImagToComplex
  Trigonometric Function : Trigonometry
  Uabc_ref : Outport  VectorParamsAs1DForOutWhenUnconnected=off
  tag scope: m=global
  wires:
  Constant1/1 -> Gain1/1
  VdVq_conv/1 -> Product1/1
  Product1/1 -> Demux1/1
  Gain1/1 -> Product/1
  Real-Imag to Complex/1 -> Complex to Magnitude-Angle/1
  Demux1/1 -> Real-Imag to Complex/1
  Demux1/2 -> Real-Imag to Complex/2
  Constant2/1 -> Add1/2
  Constant/1 -> Add1/3
  Constant3/1 -> Product/2
  Product/1 -> Product1/2
  Complex to Magnitude-Angle/2 -> Add2/1
  Add1/1 -> Add2/2
  Add2/1 -> Trigonometric Function/1
  Complex to Magnitude-Angle/1 -> [m], Product2/1
  Trigonometric Function/1 -> Product2/2
  Product2/1 -> Uabc_ref/1
  wt/1 -> Add1/1
  Constant4/1 -> Add1/4

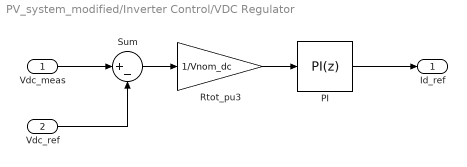
== system PV_system_modified/Inverter Control/VDC Regulator ==
  Vdc_meas : Inport  PortDimensions=1
  Vdc_ref : Inport  Port=2  PortDimensions=1
  PI : slpidlib/PID Controller  Controller=PI  Form=Parallel  TimeDomain=Discrete-time  UseExternalTs=off  SampleTime=Ts_Control  IntegratorMethod=Trapezoidal  FilterMethod=Forward Euler  ControllerParametersSource=internal  P=Kp_VDCreg  I=Ki_VDCreg  UseKiTs=off  D=0  UseExternalDerivativeSource=off  N=100  UseFilter=on  TunerSelectOption=Transfer Function Based (PID Tuner App)  InitialConditionSource=internal  InitialConditionForIntegrator=1  InitialConditionForFilter=0  DifferentiatorICPrevScaledInput=0  ExternalReset=none  TrackingMode=off  Kt=1  LimitOutput=on  SatLimitsSource=internal  UpperSaturationLimit=LimitU_VDCreg  LowerSaturationLimit=LimitL_VDCreg  LinearizeAsGain=off  AntiWindupMode=none  Kb=1  LimitIntegrator=off  UpperIntegratorSaturationLimit=inf  LowerIntegratorSaturationLimit=-inf  POutMin=[]  POutMax=[]  IOutMin=[]  IOutMax=[]  DOutMin=[]  DOutMax=[]  NOutMin=[]  NOutMax=[]  SumOutMin=[]  SumOutMax=[]  SaturationOutMin=[]  SaturationOutMax=[]  PParamMin=[]  PParamMax=[]  IParamMin=[]  IParamMax=[]  DParamMin=[]  DParamMax=[]  NParamMin=[]  NParamMax=[]  KbParamMin=[]  KbParamMax=[]  KtParamMin=[]  KtParamMax=[]  KbOutMin=[]  KbOutMax=[]  KtOutMin=[]  KtOutMax=[]  IntegratorOutMin=[]  IntegratorOutMax=[]  FilterOutMin=[]  FilterOutMax=[]  SumI1OutMin=[]  SumI1OutMax=[]  SumI2OutMin=[]  SumI2OutMax=[]  SumI3OutMin=[]  SumI3OutMax=[]  SumI4OutMin=[]  SumI4OutMax=[]  SumDOutMin=[]  SumDOutMax=[]  DifferentiatorOutMin=[]  DifferentiatorOutMax=[]  FilterDiffOutCoefMin=[]  FilterDiffOutCoefMax=[]  ReciprocalOutMin=[]  ReciprocalOutMax=[]  SumDenOutMin=[]  SumDenOutMax=[]  SumNumOutMin=[]  SumNumOutMax=[]  DivideOutMin=[]  DivideOutMax=[]  UdiffTsProdOutMin=[]  UdiffTsProdOutMax=[]  NTsProdOutMin=[]  NTsProdOutMax=[]  UintegralTsProdOutMin=[]  UintegralTsProdOutMax=[]  UngainTsProdOutMin=[]  UngainTsProdOutMax=[]  ClampingZeroOutDataTypeStr=Inherit: Inherit via back propagation  ClampingZeroOutMin=[]  ClampingZeroOutMax=[]  FilterDenConstantOutDataTypeStr=Inherit: Inherit via back propagation  FilterDenConstantOutMin=[]  FilterDenConstantOutMax=[]  PCopyOutDataTypeStr=Inherit: Inherit via back propagation  PCopyOutMin=[]  PCopyOutMax=[]  NCopyOutDataTypeStr=Inherit: Inherit via back propagation  NCopyOutMin=[]  NCopyOutMax=[]  IntegratorContinuousStateAttributes=''  IntegratorStateMustResolveToSignalObject=off  IntegratorRTWStateStorageClass=Auto  FilterContinuousStateAttributes=''  FilterStateMustResolveToSignalObject=off  FilterRTWStateStorageClass=Auto  ParallelPVariant=InternalParameters  IdealPVariant=Disabled  IVariant=InternalParameters  DVariant=Disabled  IntegratorVariant=Discrete  SatVariant=Enabled  AWVariant=Passthrough  PCopyVariant=Disabled  TRVariant=Disabled  FdbkBlocksVariant=Forward  IdealPFdbkVariant=Disabled  SatFdbkVariant=Disabled  DerivativeFilterVariant=Disabled  NVariant=Disabled  NCopyVariant=Disabled_SignalSpec  FilterICVariant=Disabled  IntegratorICVariant=InternalICs  ExternalResetVariant=Disabled  TRSumVariant=Passthrough  SumFdbkVariant=Disabled  SumVariant=Sum_PI  TsampFilterVariant=InternalTs  TsampNgainVariant=Passthrough  TsampIntegralVariant=Disabled_SignalSpec  ExternalSaturationOutDataTypeStr=Inherit: Same as second input  DerivativeSourceVariant=Disabled
  Rtot_pu3 : Gain  Gain=1/Vnom_dc  SaturateOnIntegerOverflow=on  OutDataTypeStr=Inherit: Same as input  ParamDataTypeStr=Inherit: Same as input
  Sum : Sum  Inputs=|+-
  Id_ref : Outport  InitialOutput=0  VectorParamsAs1DForOutWhenUnconnected=off
  wires:
  PI/1 -> Id_ref/1
  Rtot_pu3/1 -> PI/1
  Vdc_ref/1 -> Sum/2
  Vdc_meas/1 -> Sum/1
  Sum/1 -> Rtot_pu3/1

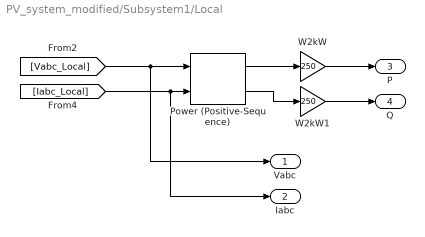
== system PV_system_modified/Subsystem1/Local ==
  Power (Positive-Sequence) : spsPowerPositiveSequenceLib/Power (Positive-Sequence)  Freq=60  Vinit=[0, 0]  Iinit=[0, 0]  Ts=Ts_Control
      settings: LibrarySourceBlock=|
      | sps_lib/Sensors and Measurements/Power
      | (Positive-Sequence)
  W2kW : Gain  Gain=250
  W2kW1 : Gain  Gain=250
  Vabc : Outport  VectorParamsAs1DForOutWhenUnconnected=off
  Iabc : Outport  Port=2  VectorParamsAs1DForOutWhenUnconnected=off
  P : Outport  Port=3  VectorParamsAs1DForOutWhenUnconnected=off
  Q : Outport  Port=4  VectorParamsAs1DForOutWhenUnconnected=off
  wires:
  Power (Positive-Sequence)/2 -> W2kW1/1
  W2kW/1 -> P/1
  Power (Positive-Sequence)/1 -> W2kW/1
  [Vabc_Local] -> Vabc/1, Power (Positive-Sequence)/1
  [Iabc_Local] -> Iabc/1, Power (Positive-Sequence)/2
  W2kW1/1 -> Q/1

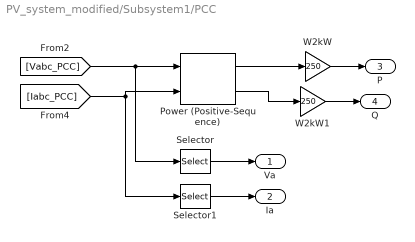
== system PV_system_modified/Subsystem1/PCC ==
  Power (Positive-Sequence) : spsPowerPositiveSequenceLib/Power (Positive-Sequence)  Freq=60  Vinit=[0, 0]  Iinit=[0, 0]  Ts=Ts_Control
      settings: LibrarySourceBlock=|
      | sps_lib/Sensors and Measurements/Power
      | (Positive-Sequence)
  Selector : Selector  InputPortWidth=3  IndexOptions=Index vector (dialog)  Indices=[1]  OutputSizes=1
  Selector1 : Selector  InputPortWidth=3  IndexOptions=Index vector (dialog)  Indices=[1]  OutputSizes=1
  W2kW : Gain  Gain=250
  W2kW1 : Gain  Gain=250
  Va : Outport  VectorParamsAs1DForOutWhenUnconnected=off
  Ia : Outport  Port=2  VectorParamsAs1DForOutWhenUnconnected=off
  P : Outport  Port=3  VectorParamsAs1DForOutWhenUnconnected=off
  Q : Outport  Port=4  VectorParamsAs1DForOutWhenUnconnected=off
  wires:
  W2kW1/1 -> Q/1
  [Iabc_PCC] -> Selector1/1, Power (Positive-Sequence)/2
  [Vabc_PCC] -> Selector/1, Power (Positive-Sequence)/1
  Power (Positive-Sequence)/1 -> W2kW/1
  W2kW/1 -> P/1
  Power (Positive-Sequence)/2 -> W2kW1/1
  Selector/1 -> Va/1
  Selector1/1 -> Ia/1

== matlab function PV_system_modified/Inverter Control/MPPT Controller using Perturbe & Observe technique  ==
  settings: updateMethod=DISCRETE  sampleTime=Ts_Control
  data: Param input; Enabled input; V input; I input; D output
function D  = PandO(Param, Enabled, V, I)

% MPPT controller based on the Perturb & Observe algorithm.

% D output = Reference for DC link voltage (Vdc_ref) 
%
% Enabled input = 1 to enable the MPPT controller
% V input = PV array terminal voltage (V)
% I input = PV array current (A)
%
% Param input:
Dinit = Param(1);  %Initial value for Vdc_ref
Dmax = Param(2);   %Maximum value for Vdc_ref
Dmin = Param(3);   %Minimum value for Vdc_ref
deltaD = Param(4); %Increment value used to increase/decrease Vdc_ref
%  

persistent Vold Pold Dold;

dataType = 'double';

if isempty(Vold)
    Vold=0;
    Pold=0;
    Dold=Dinit;
end
P= V*I;
dV= V - Vold;
dP= P - Pold;

if dP ~= 0 & Enabled ~=0
    if dP < 0
        if dV < 0
            D = Dold + deltaD;
        else
            D = Dold - deltaD;
        end
    else
        if dV < 0
            D = Dold - deltaD;
        else
            D = Dold + deltaD;
        end    
    end
else D=Dold;
end

if D >= Dmax | D<= Dmin
    D=Dold;
end

Dold=D;
Vold=V;
Pold=P;
